simulink model "mpc_block"  (R2020b)
settings: Solver=ode4  StartTime=0.0  StopTime=10.0  FixedStep=T  RelTol=1e-3
undefined symbols (not defined in the file or in its folder): mpc_ctrl_param
settings Model: Creator=vince  LastModifiedBy=vince
settings DataIOCC: ReturnWorkspaceOutputs=off

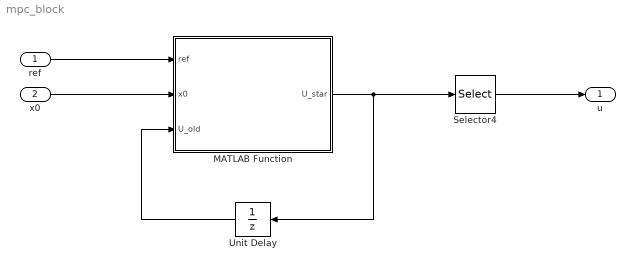
== system mpc_block ==
  ref : Inport
  x0 : Inport  Port=2
  MATLAB Function : MATLAB Function  TreatAsAtomicUnit=on
  Selector4 : Selector  InputPortWidth=mpc_ctrl_param.nu*mpc_ctrl_param.Nc  IndexOptions=Index vector (dialog)  Indices=1:mpc_ctrl_param.nu  OutputSizes=1
  Unit Delay : UnitDelay  InitialCondition=zeros(mpc_ctrl_param.nu*mpc_ctrl_param.Nc, 1)  SampleTime=mpc_ctrl_param.Ts  HasFrameUpgradeWarning=on
  u : Outport
  wires:
  ref/1 -> MATLAB Function/1(ref)
  Unit Delay/1 -> MATLAB Function/3(U_old)
  MATLAB Function/1(U_star) -> Unit Delay/1, Selector4/1
  x0/1 -> MATLAB Function/2(x0)
  Selector4/1 -> u/1

== matlab function mpc_block/MATLAB Function ==
  data: ref input; U_star output; x0 input; U_old input; mpc_ctrl_param parameter
function U_star  = mpc_optimization(ref, x0, U_old, mpc_ctrl_param)
%% Documentation
%{
    IN: x, U_old
    OUT: U*
%}


%% Prediction model
u0 = U_old(1:nu);
pred_model = model(x0, u0, Ts);


%% MPC QP design
mpc = qp_matrices(mpc_ctrl_param, pred_model, ref);


%% Objective function
H = mpc.R_bar + mpc.B_bar'*mpc.Q_bar*mpc.B_bar;
H = (H+H')/2;
f = (mpc.A_bar*x0+mpc.K_bar-mpc.REF)'*mpc.Q_bar*(mpc.B_bar);


%% Constraints
A_ineq = [-mpc.B_bar;
          mpc.B_bar;
          -eye(mpc_ctrl_param.nu*mpc_ctrl_param.Nc);
          eye(mpc_ctrl_param.nu*mpc_ctrl_param.Nc);
          -eye(mpc_ctrl_param.nu*mpc_ctrl_param.Nc);
          eye(mpc_ctrl_param.nu*mpc_ctrl_param.Nc)];

b_ineq = [-mpc.X_min + mpc.A_bar*x0 + mpc.K_bar;
          mpc.X_max - mpc.A_bar*x0 - mpc.K_bar;
          -mpc.U_min;
          mpc.U_max;
          -mpc.dU_min - U_old;
          mpc.dU_max + U_old];


%% Optimization: J(u(k)) = U(k)'*H*U(k) + f'*U(k)
coder.extrinsic('quadprog');
U_star = zeros(mpc_ctrl_param.nu*mpc_ctrl_param.Nc, 1);
U_star = quadprog(H, f, A_ineq, b_ineq, [], [], [], [], []);
